simulink model "LQI"  (R2022b)
settings: Solver=VariableStepAuto  StartTime=0.0  StopTime=10.0  RelTol=1e-3
values from neighbouring files (symbols this model uses):
  A = [0 1 ; -Ks/m -Kd/m]    [state_space_model.m]
  B = [0 ; 1/m]    [state_space_model.m]
  C = [1 0]    [state_space_model.m]
undefined symbols (not defined in the file or in its folder): Co, Kc, Ki, L
settings Model: Creator=hp  LastModifiedBy=hp

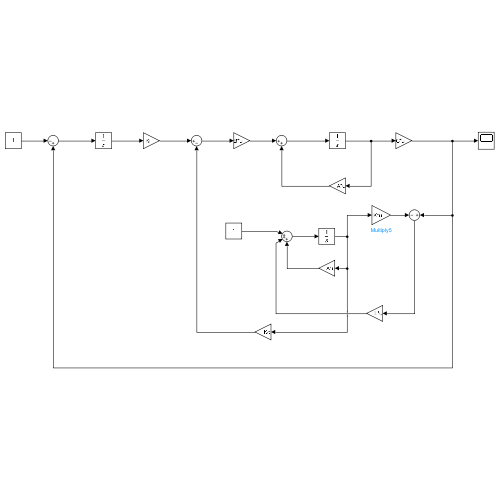
[thumbnail: Simulink's stored preview of the top-level diagram]
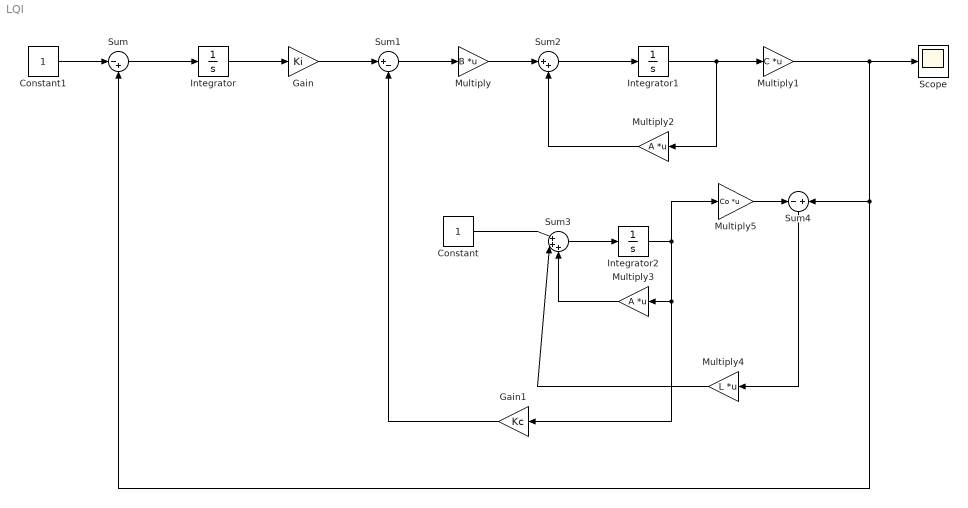
== system LQI ==
  Constant : Constant
  Constant1 : Constant
  Gain : Gain  Gain=Ki
  Gain1 : Gain  Gain=Kc
  Integrator : Integrator
  Integrator1 : Integrator
  Integrator2 : Integrator
  Multiply : Gain  Gain=B  Multiplication=Matrix(K*u)
  Multiply1 : Gain  Gain=C  Multiplication=Matrix(K*u)
  Multiply2 : Gain  Gain=A  Multiplication=Matrix(K*u)
  Multiply3 : Gain  Gain=A  Multiplication=Matrix(K*u)
  Multiply4 : Gain  Gain=L  Multiplication=Matrix(K*u)
  Multiply5 : Gain  Gain=Co  Multiplication=Matrix(K*u)
  Scope : Scope
  Sum : Sum  Inputs=|-+
  Sum1 : Sum  Inputs=|+-
  Sum2 : Sum  Inputs=|++
  Sum3 : Sum  Inputs=|+++
  Sum4 : Sum  Inputs=-+
  wires:
  Sum/1 -> Integrator/1
  Integrator/1 -> Gain/1
  Gain/1 -> Sum1/1
  Sum1/1 -> Multiply/1
  Sum2/1 -> Integrator1/1
  Integrator1/1 -> Multiply2/1, Multiply1/1
  Multiply/1 -> Sum2/1
  Constant/1 -> Sum3/1
  Sum3/1 -> Integrator2/1
  Multiply2/1 -> Sum2/2
  Multiply5/1 -> Sum4/1
  Multiply4/1 -> Sum3/2
  Gain1/1 -> Sum1/2
  Integrator2/1 -> Multiply3/1, Gain1/1, Multiply5/1
  Multiply1/1 -> Sum/2, Sum4/2, Scope/1
  Constant1/1 -> Sum/1
  Sum4/1 -> Multiply4/1
  Multiply3/1 -> Sum3/3
